simulink library "thrustCurve_ul"  (R2019a)
settings: Solver=VariableStepAuto  StartTime=0.0  StopTime=10.0  RelTol=1e-3
settings Model: Creator=John Jr  LastModifiedBy=John Jr

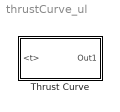
== system thrustCurve_ul ==
  "Thrust Curve " : Subsystem  mask{F_th=0, T_b=0, eta=0}
      mask prompts: F_th "Motor thrust curve [N]"
      mask Display:
      | patch([0 1 1 0], [0 0 1 1],[.8 1 1])
      | 
      | port_label('input',1,'t [s]','texmode','on')
      | 
      | port_label('output',1,'F_{th} [N]','texmode','on')

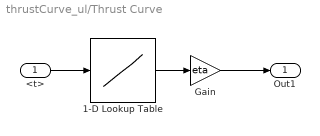
== system thrustCurve_ul/Thrust Curve  ==
  <t> : Inport
  1-D Lookup Table : Lookup_n-D  NumberOfTableDimensions=1  BreakpointsForDimension1=T_b  Table=F_th  InternalRulePriority=Speed  RndMeth=Simplest  InputSameDT=on
  Gain : Gain  Gain=eta
  Out1 : Outport
  wires:
  1-D Lookup Table/1 -> Gain/1
  <t>/1 -> 1-D Lookup Table/1
  Gain/1 -> Out1/1
